simulink model "BLT_ques_3"  (R2020a)
settings: Solver=VariableStepAuto  StartTime=0.0  StopTime=10.0  RelTol=1e-3
settings Model: Creator=DELL  LastModifiedBy=DELL

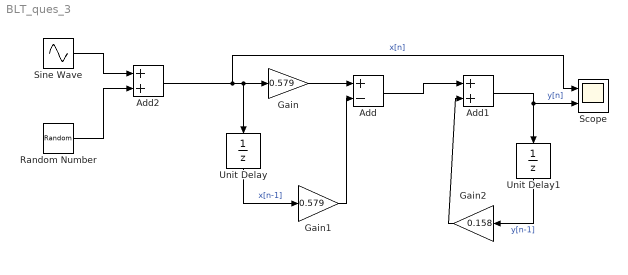
== system BLT_ques_3 ==
  Add : Sum  Inputs=+-
  Add1 : Sum
  Add2 : Sum
  Gain : Gain  Gain=0.579
  Gain1 : Gain  Gain=0.579
  Gain2 : Gain  Gain=0.158
  Random Number : RandomNumber  SampleTime=0.1
  Scope : Scope  NumInputPorts=2
  Sine Wave : Sin  Frequency=60000  SampleTime=0
  Unit Delay : UnitDelay  SampleTime=-1  HasFrameUpgradeWarning=on
  Unit Delay1 : UnitDelay  SampleTime=-1  HasFrameUpgradeWarning=on
  wires:
  Add2/1 -> Scope/1, Unit Delay/1, Gain/1  "x[n]"
  Unit Delay/1 -> Gain1/1  "x[n-1]"
  Gain1/1 -> Add/2
  Gain/1 -> Add/1
  Add/1 -> Add1/1
  Add1/1 -> Unit Delay1/1, Scope/2  "y[n]"
  Unit Delay1/1 -> Gain2/1  "y[n-1]"
  Gain2/1 -> Add1/2
  Sine Wave/1 -> Add2/1
  Random Number/1 -> Add2/2
